simulink model "Transf_1f"  (Simulink 4.00)
settings: Solver=ode23tb  StartTime=0.0  StopTime=0.1
InitFcn:
  | powericon('psbinitsys',bdroot);
libraries: powerlib2 x10, powerlib_extras x1
settings Model: SaveTime=off  SaveOutput=off  SaveFormat=Structure  LimitDataPoints=off  BlockReductionOpt=off

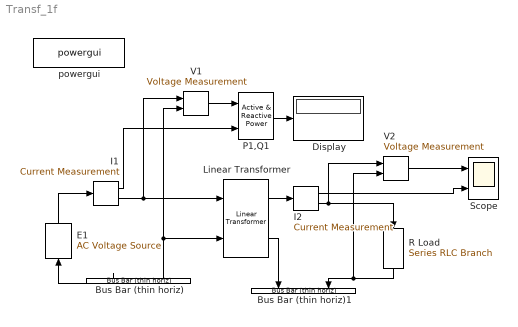
== system Transf_1f ==
  Bus Bar (thin horiz) : powerlib2/Connectors/Bus Bar (thin horiz)  Tag=PoWeRsYsTeMbLoCk  Orientation=up  input=0  output=2  PSBOutputType=111111111111111111111111111111111111111111111111111111111111111111111111111111111111
  Bus Bar (thin horiz)1 : powerlib2/Connectors/Bus Bar (thin horiz)  Tag=PoWeRsYsTeMbLoCk  Orientation=down  input=2  output=0  PSBOutputType=111111111111111111111111111111111111111111111111111111111111111111111111111111111111
  Display : Display
      settings: Format=short  Decimation=5  SampleTime=0
  E1 : powerlib2/Electrical Sources/AC Voltage Source  Tag=PoWeRsYsTeMbLoCk  Description=source block  Orientation=up  A=310  P=0  F=50  stime=0  mesure=None  PSBOutputType=1
  I1 : powerlib2/Measurements/Current Measurement  Tag=PoWeRsYsTeMmEaSuReMeNt  PSBOutputType=01  PSBequivalent=0
  I2 : powerlib2/Measurements/Current Measurement  Tag=PoWeRsYsTeMmEaSuReMeNt  PSBOutputType=01  PSBequivalent=0
  Linear Transformer : powerlib2/Elements/Linear Transformer  Tag=PoWeRsYsTeMbLoCk  a=[250 50]  b=[220 0.02 0.08]  c=[100 0.02 0.08]  d=[0]  e=[500 500]  mesure=None  PSBOutputType=1111
  P1,Q1 : powerlib_extras/Measurements/Active & Reactive Power  f1=50
  R Load : powerlib2/Elements/Series RLC Branch  Tag=PoWeRsYsTeMbLoCk  Orientation=down  a=50  b=0  c=inf  mesure=None  PSBOutputType=1
  Scope : Scope  NumInputPorts=2
      settings: TimeRange=auto  YMin=-100~-5  YMax=100~5  SaveToWorkspace=off  SaveName=ScopeData  MaxDataPoints=5000
  V1 : powerlib2/Measurements/Voltage Measurement  Tag=PoWeRsYsTeMmEaSuReMeNt  PSBOutputType=0  PSBequivalent=0
  V2 : powerlib2/Measurements/Voltage Measurement  Tag=PoWeRsYsTeMmEaSuReMeNt  PSBOutputType=0  PSBequivalent=1
  powergui : powerlib2/powergui  matfilesaved=off  Frange=logspace(0,3,50)  Ylog=off  Xlog=off  save=off  variable=ZData  display=off
  wires:
  E1/1 -> I1/1
  I1/2 -> Linear Transformer/1, V1/1
  Bus Bar (thin horiz)/1 -> E1/1
  Bus Bar (thin horiz)/2 -> Linear Transformer/2, V1/2
  Linear Transformer/1 -> I2/1
  Linear Transformer/2 -> Bus Bar (thin horiz)1/1
  V1/1 -> P1,Q1/1
  I1/1 -> P1,Q1/2
  P1,Q1/1 -> Display/1
  V2/1 -> Scope/1
  I2/1 -> Scope/2
  I2/2 -> R Load/1, V2/1
  R Load/1 -> Bus Bar (thin horiz)1/2, V2/2
